simulink model "AIE_HLS_clipping"  (R2023a)
settings: Solver=VariableStepAuto  StartTime=0.0  StopTime=inf  RelTol=1e-3
InitFcn:
  | load filter_coeffs.mat
  | LPF = round(LPF * 2^15)
undefined symbols (not defined in the file): None, S, vsva2197, xcvc1902
libraries: aieBasic x3, aieDSP x2, aieUtilities x2, dspfdesign x1, vmcUtilities x1, hlsBasic x1
settings Model: Creator=abehbood  LastModifiedBy=robg
settings DebuggingCC: UnconnectedInputMsg=warning  UnconnectedOutputMsg=warning  UnconnectedLineMsg=warning
settings ModelReferenceCC: EnableRefExpFcnMdlSchedulingChecks=on
settings RTWCC: DLArmComputeVersion=19.05

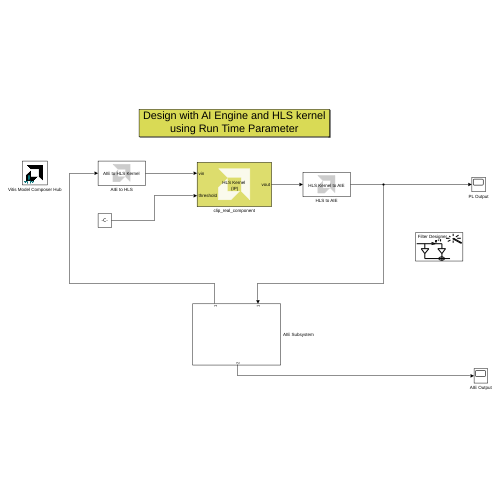
[thumbnail: Simulink's stored preview of the top-level diagram]
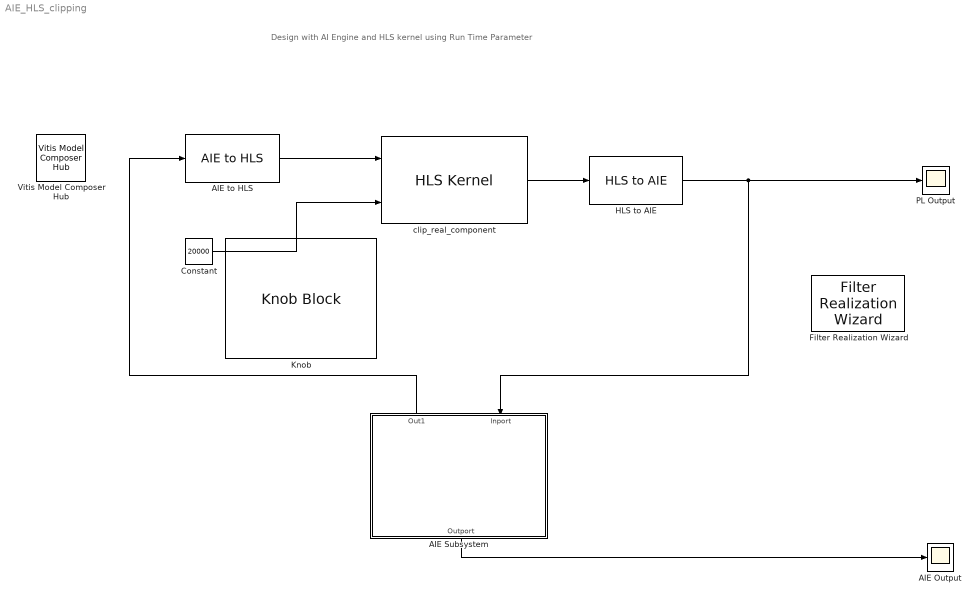
== system AIE_HLS_clipping ==
  note: Design with AI Engine and HLS kernel
      | using Run Time Parameter
  AIE Output : Scope
  AIE Subsystem : Subsystem
      settings: PortSchema="{\"entries\":[{\"content\":{\"sides\":[{\"content\":{\"connectorIds\":[\"Out2\"]},\"type\":\"ConnectorPlacement.EquallySpacedRectSide\",\"uuid\":\"600439e9-73c3-433c-a4a4-c36b72988664\"},{\"content\":{\"connectorIds\":[\"Out1\",\"In1\"],\"side\":\"RIGHT\"},\"type\":\"ConnectorPlacement.EquallySpacedRectSide\",\"uuid\":\"c5ca9a85-0742-44d8-b50a-7698103ab251\"},{\"content\":{\"connectorIds\":[],\"side\":\"TOP\"},\"type\":\"ConnectorPlacement.EquallySpacedRectSide\",\"uuid\":\"fb61f941-2da5-44dc-abf4-df4618bee3ad\"},{\"content\":{\"connectorIds\":[],\"side\":\"BOTTOM\"},\"type\":\"ConnectorPlacement.EquallySpacedRectSide\",\"uuid\":\"5a66f69a-5526-4d5e-a2d5-c31759d47fa6\"}]},\"type\":\"ConnectorPlacement.EquallySpacedConnector\",\"uuid\":\"81997a57-f7dc-4123-9425-e160d8e12fe0\"}],\"packageUris\":[\"http://schema.mathworks.com/mf0/Connector/R2020b\"],\"version\":\"1.0\"}"
  AIE to HLS : aieUtilities/AIE to HLS  OutputType=cint16  OutputSize=32
  Constant : Constant  Value=20000  OutDataTypeStr=int32  SampleTime=-1
  Filter Realization Wizard : dspfdesign/Filter Realization Wizard
  HLS to AIE : aieUtilities/HLS to AIE  OutputType=cint16  OutputSize=32
  Knob : KnobBlock  LabelPosition=Hide  ScaleMin=20000  ScaleMax=32767
  PL Output : Scope
  Vitis Model Composer Hub : vmcUtilities/Vitis Model Composer Hub  Tag=genX  CodeGeneration=off  SubsystemName=AIE Subsystem  StartColumn=1  NumberOfColumns=1  TargetDirectory=./code  exportDesign=off  analyzeDesign=off  validateDesignOnHw=off  ExportType=AI Engines  IpVendor=xilinx.com  IpLibrary=hls  IpVersion=1.0  IpHWLanguage=Verilog  AieCompilerOptions={}  AieSimulatorOptions={}  CreateTestbench=on  TestbenchStackSize=10  RunRtlSim=off  RunCSim=off  RunAieSim=on  AieSimTimeout=5000  RunAieSimProfiling=off  LaunchVitisAnalyzer=off  PlotOutput=off  RunX86Sim=off  X86SimTimeout=10  GenHwImage=off  GenLibadfXo=off  GenHwValidationCode=off  PlatformType=Not Specified  HwSystemType=Baremetal  HwValidationTarget=hw  ProjDevice=xcvc1902-vsva2197-1LP-e-S  ProjDevicePart=xcvc1902-vsva2197-1LP-e-S  AIEType=AIE  SamplePeriod=-1  ClockFrequency=200  DataPathParallelism=1  xilinxfamily=Kintex7  part=xc7k325t  speed=-3  package=fbg676  directory=./netlist  testbench=off  incr_netlist=off  synthesis_tool=Vivado  clock_wrapper=Clock Enables  dbl_ovrd=According to Block Masks  dcm_input_clock_period=10  sysclk_period=10  simulink_period=1  eval_field=0  LogFileName=''  NThreads=4
  clip_real_component : hlsBasic/HLS Kernel  PortNames={'return'; 'vin'; 'threshold'; 'vout'}  PortSerializedTypes={'{Bv}'; '{R{Thls::stream{2{t{Tstd::complex{1{t{Bi16}}}}}{t{}0}}}}'; '{Bi32}'; '{R{Thls::stream{2{t{Tstd::complex{1{t{Bi16}}}}}{t{}0}}}}'}  FunctionTemplateSpecKind=none  FunctionTemplateParamNames={}  FunctionTemplateParamKinds={}  FunctionTemplateParamTypes={}  FunctionTemplateParamValues={}  PortSynchronicities={'auto'; 'sync'; 'auto'}  PortSignalSizes={0.000000000000000000e+00; 0.000000000000000000e+00; 3.200000000000000000e+01}  PortParameterValues={}  FunctionTemplateParams={}  FunctionTemplateParamsEnables={}  FunctionTemplateParamsVisible=off  FunctionDeclTypeOptions=C[1 1]@t7@<empty>  PortAttributesTable={ 'Input', 'vin', 'hls::stream< std::complex< int16 >, 0 > &', '', ''; 'Input', 'threshold', 'int32', 'async', ''; 'Output', 'vout', 'hls::stream< std::complex< int16 >, 0 > &', '', '32' }  PortAttributesEnablement={'off', 'off', 'off', 'off', 'off';'off', 'off', 'off', 'on', 'off';'off', 'off', 'off', 'off', 'on'}  PortParametersTable={}  SampleTime=-1  PortDirectionTable={ 'vin', 'hls::stream< std::complex< int16 >, 0 > &', 'Input'; 'threshold', 'int32', 'Input'; 'vout', 'hls::stream< std::complex< int16 >, 0 > &', 'Output' }  PortDirectionTabVisible=on  ArgDirections={1.000000000000000000e+00; 1.000000000000000000e+00; 2.000000000000000000e+00}  ArgInterfaceTypes={}  FunctionIndex=1  FormalArgDecls={'hls::stream< std::complex< int16 >, 0 > & vin', 'int32 threshold', 'hls::stream< std::complex< int16 >, 0 > & vout'}  SimLibPath=''  FunctionTabVisible=on  FunctionDescription=void clipper(hls::stream< std::complex< int16 >, 0 > & vin, int32 threshold, hls::stream< std::complex< int16 >, 0 > & vout)  blockJsonConstraints=[]  deprecateConstraints=0  KernelHeaderFile=src/clipper.h  KernelFunction=clipper  KernelFunctionSelect=<empty>  KernelSourceFile=src/clipper.cpp  KernelSearchPaths={}  PreProcOptions={}
  wires:
  AIE to HLS/1 -> clip_real_component/1
  Constant/1 -> clip_real_component/2
  clip_real_component/1 -> HLS to AIE/1
  AIE Subsystem/1(Out1) -> AIE to HLS/1
  AIE Subsystem/2(Outport) -> AIE Output/1
  HLS to AIE/1 -> AIE Subsystem/1(Inport), PL Output/1

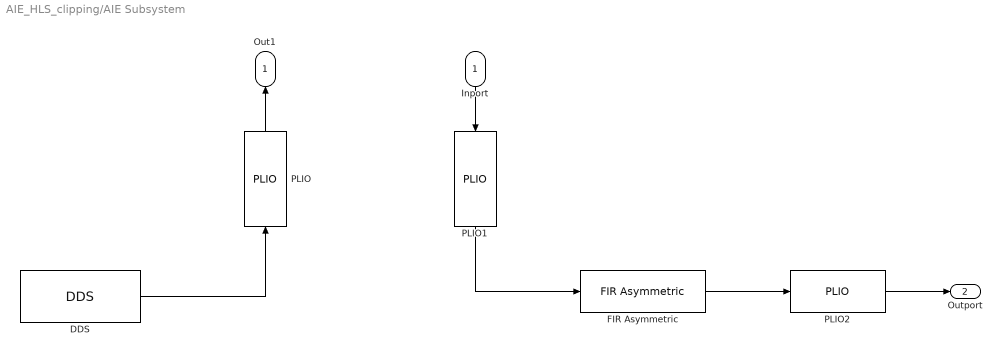
== system AIE_HLS_clipping/AIE Subsystem ==
  Inport : Inport
  DDS : aieDSP/DDS  data_type=cint16  output_window_size=32  ssr=1  USE_PHASE_RELOAD=off  phase_increment=2^25  rnd_mode=Floor  sat_mode=0-None  vmc_sample_time=3.0518e-05  AIE_VARIANT=1  blockJsonConstraints=[]  blockJsonConstraintsInternal=[]  spec=vmc_dds.json  SerializedMaskParamNames=[]  SerializedMaskParamValues=[]  SerializedMaskParamVisibilities=[]  block_type=DDS  SerializedMaskParamDataypes=typename|uint|uint|bool|uint|uint|uint|double|uint  SerializedMaskParamEnumStrArr=0|0|0|0|0|Floor,Ceiling,Round to positive infinity,Round to negative infinity,Round symmetrical to infinity,Round symmetrical to zero,Round convergent to even,Round convergent to odd|0-None,1-Asymmetric,3-Symmetric|0|0  SerializedMaskParamEnumValArr=0|0|0|0|0|0,1,2,3,4,5,6,7|0,1,3|0|0  SerializedMaskParamVectorArr=0|0|0|0|0|0|0|0|0
  FIR Asymmetric : aieDSP/FIR Asymmetric  data_type=cint16  coef_type=int16  use_coeff_reload=off  num_outputs=off  coeff=LPF  fir_length=32  input_window_size=32  shift_val=16  rnd_mode=Round to positive infinity  sat_mode=0-None  casc_length=1  AIE_VARIANT=1  blockJsonConstraints=[]  blockJsonConstraintsInternal=[]  spec=vmc_fir_sr_asym.json  SerializedMaskParamNames=[]  SerializedMaskParamValues=[]  SerializedMaskParamVisibilities=[]  block_type=FIR Asymmetric  SerializedMaskParamDataypes=typename|typename|bool|bool|coef_type|uint|uint|uint|uint|uint|uint|uint  SerializedMaskParamEnumStrArr=0|0|0|0|0|0|0|0|Floor,Ceiling,Round to positive infinity,Round to negative infinity,Round symmetrical to infinity,Round symmetrical to zero,Round convergent to even,Round convergent to odd|0-None,1-Asymmetric,3-Symmetric|0|0  SerializedMaskParamEnumValArr=0|0|0|0|0|0|0|0|0,1,2,3,4,5,6,7|0,1,3|0|0  SerializedMaskParamVectorArr=0|0|0|0|1|0|0|0|0|0|0|0
  PLIO : aieBasic/PLIO  PlioWidth=auto  PlioFreqSpec=off  PlioFreq=250  ColLocation=0  channel=0  blockJsonConstraints=[]  deprecateConstraints=0
  PLIO1 : aieBasic/PLIO  PlioWidth=auto  PlioFreqSpec=off  PlioFreq=250  ColLocation=0  channel=0  blockJsonConstraints=[]  deprecateConstraints=0
  PLIO2 : aieBasic/PLIO  PlioWidth=auto  PlioFreqSpec=off  PlioFreq=250  ColLocation=0  channel=0  blockJsonConstraints=[]  deprecateConstraints=0
  Out1 : Outport
  Outport : Outport  Port=2
  wires:
  DDS/1 -> PLIO/1
  PLIO/1 -> Out1/1
  FIR Asymmetric/1 -> PLIO2/1
  PLIO1/1 -> FIR Asymmetric/1
  PLIO2/1 -> Outport/1
  Inport/1 -> PLIO1/1
